simulink model "SC_Lab3_Variant3"  (R2025b)
settings: Solver=ode45  StartTime=0.0  StopTime=1  RelTol=1e-3
(part 2 of 2)

== matlab function SC_Lab3_Variant3/SensorlessCore ==
  data: ia input; dia output; ib input; omega input; theta input; zid input; ziq input; zw input; z1a input; z1b input; z2a input; z2b input; zg input; zm1 input; zm2 input; eta1h input; eta2h input; chi1 input; chi2 input; wref input; tau_L input; sensorless_mode input; dib output; domega output; dtheta output; dzid output; dziq output; dzw output; dz1a output; dz1b output; dz2a output; dz2b output; dzg output; dzm1 output; dzm2 output; deta1h output; deta2h output; dchi1 output; dchi2 output; wref_out output; tauL_out output; open_e_omega output; eta1_err output; eta2_err output; lambda_a_err output; lambda_b_err output; theta_err output; omega_err output; closed_e_omega output; closed_theta_err output; closed_omega_err output
function [dia, dib, domega, dtheta, dzid, dziq, dzw, dz1a, dz1b, dz2a, dz2b, dzg, dzm1, dzm2, deta1h, deta2h, dchi1, dchi2, wref_out, tauL_out, open_e_omega, eta1_err, eta2_err, lambda_a_err, lambda_b_err, theta_err, omega_err, closed_e_omega, closed_theta_err, closed_omega_err] = fcn(ia, ib, omega, theta, zid, ziq, zw, z1a, z1b, z2a, z2b, zg, zm1, zm2, eta1h, eta2h, chi1, chi2, wref, tau_L, sensorless_mode)
                                                                                                                                                                                                                                                                                                                                                                                                                          L = 0.033;                                                                                                                                                                                                                                                                                                                                                                                                                 
                                                                                                                                                                                                                                                                                                                                                                                                                          R = 5.3;                                                                                                                                                                                                                                                                                                                                                                                                                   
                                                                                                                                                                                                                                                                                                                                                                                                                          Jm = 0.0006;                                                                                                                                                                                                                                                                                                                                                                                                               
                                                                                                                                                                                                                                                                                                                                                                                                                          np = 5;                                                                                                                                                                                                                                                                                                                                                                                                                    
                                                                                                                                                                                                                                                                                                                                                                                                                          lambda_m = 0.16;                                                                                                                                                                                                                                                                                                                                                                                                           
                                                                                                                                                                                                                                                                                                                                                                                                                          B = 0;                                                                                                                                                                                                                                                                                                                                                                                                                     
                                                                                                                                                                                                                                                                                                                                                                                                                          kp_i = 18;                                                                                                                                                                                                                                                                                                                                                                                                                 
                                                                                                                                                                                                                                                                                                                                                                                                                          ki_i = 1400;                                                                                                                                                                                                                                                                                                                                                                                                               
                                                                                                                                                                                                                                                                                                                                                                                                                          kp_w = 0.36;                                                                                                                                                                                                                                                                                                                                                                                                               
                                                                                                                                                                                                                                                                                                                                                                                                                          ki_w = 18;                                                                                                                                                                                                                                                                                                                                                                                                                 
                                                                                                                                                                                                                                                                                                                                                                                                                          iq_limit = 25;                                                                                                                                                                                                                                                                                                                                                                                                             
                                                                                                                                                                                                                                                                                                                                                                                                                          v_limit = 120;                                                                                                                                                                                                                                                                                                                                                                                                             
                                                                                                                                                                                                                                                                                                                                                                                                                          alpha = 250;                                                                                                                                                                                                                                                                                                                                                                                                               
                                                                                                                                                                                                                                                                                                                                                                                                                          gamma = 2.5;                                                                                                                                                                                                                                                                                                                                                                                                               
                                                                                                                                                                                                                                                                                                                                                                                                                          pll_kp = 252;                                                                                                                                                                                                                                                                                                                                                                                                              
                                                                                                                                                                                                                                                                                                                                                                                                                          pll_ki = 32400;                                                                                                                                                                                                                                                                                                                                                                                                            
                                                                                                                                                                                                                                                                                                                                                                                                                          period = 2*pi/np;                                                                                                                                                                                                                                                                                                                                                                                                          
                                                                                                                                                                                                                                                                                                                                                                                                                          theta_e = np * theta;                                                                                                                                                                                                                                                                                                                                                                                                      
                                                                                                                                                                                                                                                                                                                                                                                                                          x1 = lambda_m*cos(theta_e);                                                                                                                                                                                                                                                                                                                                                                                                
                                                                                                                                                                                                                                                                                                                                                                                                                          x2 = lambda_m*sin(theta_e);                                                                                                                                                                                                                                                                                                                                                                                                
                                                                                                                                                                                                                                                                                                                                                                                                                          m1 = z1a - L*ia - R*z2a;                                                                                                                                                                                                                                                                                                                                                                                                   
                                                                                                                                                                                                                                                                                                                                                                                                                          m2 = z1b - L*ib - R*z2b;                                                                                                                                                                                                                                                                                                                                                                                                   
                                                                                                                                                                                                                                                                                                                                                                                                                          g = -(m1*m1 + m2*m2);                                                                                                                                                                                                                                                                                                                                                                                                      
                                                                                                                                                                                                                                                                                                                                                                                                                          y_f = alpha*(g - zg);                                                                                                                                                                                                                                                                                                                                                                                                      
                                                                                                                                                                                                                                                                                                                                                                                                                          q1_f = 2*alpha*(m1 - zm1);                                                                                                                                                                                                                                                                                                                                                                                                 
                                                                                                                                                                                                                                                                                                                                                                                                                          q2_f = 2*alpha*(m2 - zm2);                                                                                                                                                                                                                                                                                                                                                                                                 
                                                                                                                                                                                                                                                                                                                                                                                                                          dzg = alpha*(g - zg);                                                                                                                                                                                                                                                                                                                                                                                                      
                                                                                                                                                                                                                                                                                                                                                                                                                          dzm1 = alpha*(m1 - zm1);                                                                                                                                                                                                                                                                                                                                                                                                   
                                                                                                                                                                                                                                                                                                                                                                                                                          dzm2 = alpha*(m2 - zm2);                                                                                                                                                                                                                                                                                                                                                                                                   
                                                                                                                                                                                                                                                                                                                                                                                                                          eps_reg = y_f - q1_f*eta1h - q2_f*eta2h;                                                                                                                                                                                                                                                                                                                                                                                   
                                                                                                                                                                                                                                                                                                                                                                                                                          deta1h = gamma*q1_f*eps_reg;                                                                                                                                                                                                                                                                                                                                                                                               
                                                                                                                                                                                                                                                                                                                                                                                                                          deta2h = gamma*q2_f*eps_reg;                                                                                                                                                                                                                                                                                                                                                                                               
                                                                                                                                                                                                                                                                                                                                                                                                                          x1h = m1 + eta1h;                                                                                                                                                                                                                                                                                                                                                                                                          
                                                                                                                                                                                                                                                                                                                                                                                                                          x2h = m2 + eta2h;                                                                                                                                                                                                                                                                                                                                                                                                          
                                                                                                                                                                                                                                                                                                                                                                                                                          theta_raw = atan2(x2h, x1h)/np;                                                                                                                                                                                                                                                                                                                                                                                            
                                                                                                                                                                                                                                                                                                                                                                                                                          theta_pll_err = mod(theta_raw - chi1 + period/2, period) - period/2;                                                                                                                                                                                                                                                                                                                                                       
                                                                                                                                                                                                                                                                                                                                                                                                                          omega_hat = pll_kp*theta_pll_err + pll_ki*chi2;                                                                                                                                                                                                                                                                                                                                                                            
                                                                                                                                                                                                                                                                                                                                                                                                                          dchi1 = omega_hat;                                                                                                                                                                                                                                                                                                                                                                                                         
                                                                                                                                                                                                                                                                                                                                                                                                                          dchi2 = theta_pll_err;                                                                                                                                                                                                                                                                                                                                                                                                     
                                                                                                                                                                                                                                                                                                                                                                                                                          theta_ctrl = theta;                                                                                                                                                                                                                                                                                                                                                                                                        
                                                                                                                                                                                                                                                                                                                                                                                                                          if sensorless_mode > 0.5                                                                                                                                                                                                                                                                                                                                                                                                   
                                                                                                                                                                                                                                                                                                                                                                                                                              theta_ctrl = chi1;                                                                                                                                                                                                                                                                                                                                                                                                     
                                                                                                                                                                                                                                                                                                                                                                                                                          end                                                                                                                                                                                                                                                                                                                                                                                                                        
                                                                                                                                                                                                                                                                                                                                                                                                                          theta_e_ctrl = np*theta_ctrl;                                                                                                                                                                                                                                                                                                                                                                                              
                                                                                                                                                                                                                                                                                                                                                                                                                          c = cos(theta_e_ctrl);                                                                                                                                                                                                                                                                                                                                                                                                     
                                                                                                                                                                                                                                                                                                                                                                                                                          s = sin(theta_e_ctrl);                                                                                                                                                                                                                                                                                                                                                                                                     
                                                                                                                                                                                                                                                                                                                                                                                                                          id = c*ia + s*ib;                                                                                                                                                                                                                                                                                                                                                                                                          
                                                                                                                                                                                                                                                                                                                                                                                                                          iq = -s*ia + c*ib;                                                                                                                                                                                                                                                                                                                                                                                                         
                                                                                                                                                                                                                                                                                                                                                                                                                          wref_out = wref;                                                                                                                                                                                                                                                                                                                                                                                                           
                                                                                                                                                                                                                                                                                                                                                                                                                          tauL_out = tau_L;                                                                                                                                                                                                                                                                                                                                                                                                          
                                                                                                                                                                                                                                                                                                                                                                                                                          closed_e_omega = wref - omega;                                                                                                                                                                                                                                                                                                                                                                                             
                                                                                                                                                                                                                                                                                                                                                                                                                          iq_ref = kp_w*closed_e_omega + ki_w*zw;                                                                                                                                                                                                                                                                                                                                                                                    
                                                                                                                                                                                                                                                                                                                                                                                                                          if iq_ref > iq_limit                                                                                                                                                                                                                                                                                                                                                                                                       
                                                                                                                                                                                                                                                                                                                                                                                                                              iq_ref = iq_limit;                                                                                                                                                                                                                                                                                                                                                                                                     
                                                                                                                                                                                                                                                                                                                                                                                                                          elseif iq_ref < -iq_limit                                                                                                                                                                                                                                                                                                                                                                                                  
                                                                                                                                                                                                                                                                                                                                                                                                                              iq_ref = -iq_limit;                                                                                                                                                                                                                                                                                                                                                                                                    
                                                                                                                                                                                                                                                                                                                                                                                                                          end                                                                                                                                                                                                                                                                                                                                                                                                                        
                                                                                                                                                                                                                                                                                                                                                                                                                          e_id = -id;                                                                                                                                                                                                                                                                                                                                                                                                                
                                                                                                                                                                                                                                                                                                                                                                                                                          e_iq = iq_ref - iq;                                                                                                                                                                                                                                                                                                                                                                                                        
                                                                                                                                                                                                                                                                                                                                                                                                                          vd = kp_i*e_id + ki_i*zid - np*omega*L*iq;                                                                                                                                                                                                                                                                                                                                                                                 
                                                                                                                                                                                                                                                                                                                                                                                                                          vq = kp_i*e_iq + ki_i*ziq + np*omega*(L*id + lambda_m);                                                                                                                                                                                                                                                                                                                                                                    
                                                                                                                                                                                                                                                                                                                                                                                                                          va = c*vd - s*vq;                                                                                                                                                                                                                                                                                                                                                                                                          
                                                                                                                                                                                                                                                                                                                                                                                                                          vb = s*vd + c*vq;                                                                                                                                                                                                                                                                                                                                                                                                          
                                                                                                                                                                                                                                                                                                                                                                                                                          vnorm = sqrt(va*va + vb*vb);                                                                                                                                                                                                                                                                                                                                                                                               
                                                                                                                                                                                                                                                                                                                                                                                                                          if vnorm > v_limit                                                                                                                                                                                                                                                                                                                                                                                                         
                                                                                                                                                                                                                                                                                                                                                                                                                              scale = v_limit / vnorm;                                                                                                                                                                                                                                                                                                                                                                                               
                                                                                                                                                                                                                                                                                                                                                                                                                              va = va*scale;                                                                                                                                                                                                                                                                                                                                                                                                         
                                                                                                                                                                                                                                                                                                                                                                                                                              vb = vb*scale;                                                                                                                                                                                                                                                                                                                                                                                                         
                                                                                                                                                                                                                                                                                                                                                                                                                          end                                                                                                                                                                                                                                                                                                                                                                                                                        
                                                                                                                                                                                                                                                                                                                                                                                                                          ct = cos(theta_e);                                                                                                                                                                                                                                                                                                                                                                                                         
                                                                                                                                                                                                                                                                                                                                                                                                                          st = sin(theta_e);                                                                                                                                                                                                                                                                                                                                                                                                         
                                                                                                                                                                                                                                                                                                                                                                                                                          dia = (-R*ia + va + lambda_m*np*omega*st) / L;                                                                                                                                                                                                                                                                                                                                                                             
                                                                                                                                                                                                                                                                                                                                                                                                                          dib = (-R*ib + vb - lambda_m*np*omega*ct) / L;                                                                                                                                                                                                                                                                                                                                                                             
                                                                                                                                                                                                                                                                                                                                                                                                                          tau_e = np*lambda_m*(-ia*st + ib*ct);                                                                                                                                                                                                                                                                                                                                                                                      
                                                                                                                                                                                                                                                                                                                                                                                                                          domega = (-B*omega + tau_e - tau_L)/Jm;                                                                                                                                                                                                                                                                                                                                                                                    
                                                                                                                                                                                                                                                                                                                                                                                                                          dtheta = omega;                                                                                                                                                                                                                                                                                                                                                                                                            
                                                                                                                                                                                                                                                                                                                                                                                                                          dzid = e_id;                                                                                                                                                                                                                                                                                                                                                                                                               
                                                                                                                                                                                                                                                                                                                                                                                                                          dziq = e_iq;                                                                                                                                                                                                                                                                                                                                                                                                               
                                                                                                                                                                                                                                                                                                                                                                                                                          dzw = closed_e_omega;                                                                                                                                                                                                                                                                                                                                                                                                      
                                                                                                                                                                                                                                                                                                                                                                                                                          dz1a = va;                                                                                                                                                                                                                                                                                                                                                                                                                 
                                                                                                                                                                                                                                                                                                                                                                                                                          dz1b = vb;                                                                                                                                                                                                                                                                                                                                                                                                                 
                                                                                                                                                                                                                                                                                                                                                                                                                          dz2a = ia;                                                                                                                                                                                                                                                                                                                                                                                                                 
                                                                                                                                                                                                                                                                                                                                                                                                                          dz2b = ib;                                                                                                                                                                                                                                                                                                                                                                                                                 
                                                                                                                                                                                                                                                                                                                                                                                                                          eta1_err = lambda_m - eta1h;                                                                                                                                                                                                                                                                                                                                                                                               
                                                                                                                                                                                                                                                                                                                                                                                                                          eta2_err = -eta2h;                                                                                                                                                                                                                                                                                                                                                                                                         
                                                                                                                                                                                                                                                                                                                                                                                                                          lambda_a = L*ia + x1;                                                                                                                                                                                                                                                                                                                                                                                                      
                                                                                                                                                                                                                                                                                                                                                                                                                          lambda_b = L*ib + x2;                                                                                                                                                                                                                                                                                                                                                                                                      
                                                                                                                                                                                                                                                                                                                                                                                                                          lambda_a_hat = L*ia + x1h;                                                                                                                                                                                                                                                                                                                                                                                                 
                                                                                                                                                                                                                                                                                                                                                                                                                          lambda_b_hat = L*ib + x2h;                                                                                                                                                                                                                                                                                                                                                                                                 
                                                                                                                                                                                                                                                                                                                                                                                                                          lambda_a_err = lambda_a - lambda_a_hat;                                                                                                                                                                                                                                                                                                                                                                                    
                                                                                                                                                                                                                                                                                                                                                                                                                          lambda_b_err = lambda_b - lambda_b_hat;                                                                                                                                                                                                                                                                                                                                                                                    
                                                                                                                                                                                                                                                                                                                                                                                                                          theta_err = mod(theta - chi1 + period/2, period) - period/2;                                                                                                                                                                                                                                                                                                                                                               
                                                                                                                                                                                                                                                                                                                                                                                                                          omega_err = omega - omega_hat;                                                                                                                                                                                                                                                                                                                                                                                             
                                                                                                                                                                                                                                                                                                                                                                                                                          open_e_omega = wref - omega;                                                                                                                                                                                                                                                                                                                                                                                               
                                                                                                                                                                                                                                                                                                                                                                                                                          closed_theta_err = theta_err;                                                                                                                                                                                                                                                                                                                                                                                              
                                                                                                                                                                                                                                                                                                                                                                                                                          closed_omega_err = omega_err;
